simulink model "split_range_control"  (Simulink 3.00)
libraries: mathlib x6, analoglib x2, execlib x1, reglib x1, arclib x1

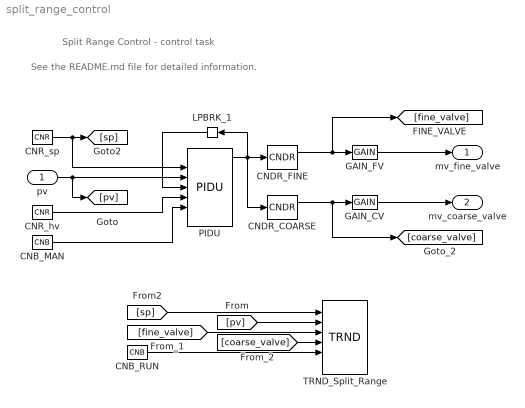
== system split_range_control ==
  note: See the README.md file for detailed information.
  note: Split Range Control - control task
  pv : Inport  Port=1
  CNB_MAN : mathlib/CNB  YCN=off
  CNB_RUN : mathlib/CNB  YCN=on
  CNDR_COARSE : analoglib/CNDR  n=2  SATF=on  up=[ 0.2, 1.0]  yp=[ 0, 1.0]
  CNDR_FINE : analoglib/CNDR  n=2  SATF=on  up=[ 0, 0.2]  yp=[ 0, 1.0]
  CNR_hv : mathlib/CNR  ycn=0.1
  CNR_sp : mathlib/CNR  ycn=0
  GAIN_CV : mathlib/GAIN  k=0.8
  GAIN_FV : mathlib/GAIN  k=0.2
  LPBRK_1 : execlib/LPBRK  Orientation=left
  PIDU : reglib/PIDU  irtype=7: PID  RACT=off  k=0.6  ti=4  td=1  nd=10  b=1  c=0  tt=1  hilim=1  lolim=0  dz=0  icotype=1: Analog
  TRND_Split_Range : arclib/TRND  n=4  l=1000  btype=8: Double  ptype1=1: Store  ptype2=1: Store  ptype3=1: Store  ptype4=1: Store  pfac=1  afac=0  arc=0  id=1  Title=Trend Title  timesrc=1
  mv_fine_valve : Outport  Port=1
  mv_coarse_valve : Outport  Port=2
  wires:
  CNB_MAN/1 -> PIDU/6
  CNB_RUN/1 -> TRND_Split_Range/5
  CNDR_COARSE/1 -> GAIN_CV/1, [coarse_valve]
  CNDR_FINE/1 -> [fine_valve], GAIN_FV/1
  CNR_hv/1 -> PIDU/5
  CNR_sp/1 -> [sp], PIDU/2
  [pv] -> TRND_Split_Range/2
  [sp] -> TRND_Split_Range/1
  [fine_valve] -> TRND_Split_Range/3
  [coarse_valve] -> TRND_Split_Range/4
  GAIN_CV/1 -> mv_coarse_valve/1
  GAIN_FV/1 -> mv_fine_valve/1
  LPBRK_1/1 -> PIDU/4
  PIDU/1 -> CNDR_COARSE/1, CNDR_FINE/1, LPBRK_1/1
  pv/1 -> [pv], PIDU/3
